simulink model "manipulator_dae"  (R2018b)
settings: Solver=VariableStepAuto  StartTime=0.0  StopTime=10.0  RelTol=1e-3
values from neighbouring files (symbols this model uses):
  alpha_rel = 60*pi/180    (= 1.0471975512)    [parameters.m]
  kp1 = 160    [parameters.m]
  kp2 = 60    [parameters.m]
  kv1 = 11    [parameters.m]
  kv2 = 1.1    [parameters.m]
  rad_deg = 180/pi    (= 57.2957795131)    [parameters.m]
undefined symbols (not defined in the file or in its folder): sys_phdae
settings Model: Creator=a.brugnoli  LastModifiedBy=a.brugnoli

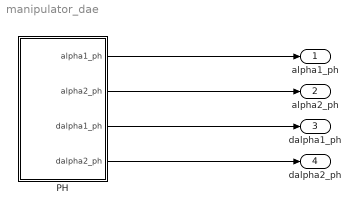
== system manipulator_dae ==
  PH : Subsystem
  alpha1_ph : Outport
  alpha2_ph : Outport  Port=2
  dalpha1_ph : Outport  Port=3
  dalpha2_ph : Outport  Port=4
  wires:
  PH/1(alpha1_ph) -> alpha1_ph/1
  PH/2(alpha2_ph) -> alpha2_ph/1
  PH/4(dalpha2_ph) -> dalpha2_ph/1
  PH/3(dalpha1_ph) -> dalpha1_ph/1

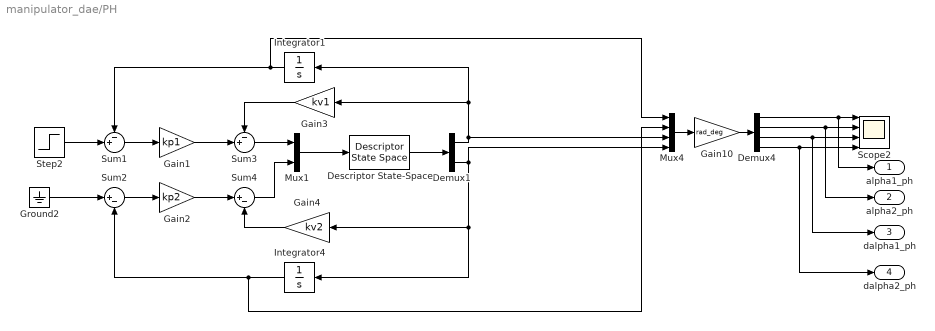
== system manipulator_dae/PH ==
  Demux1 : Demux  Outputs=2
  Demux4 : Demux
  Descriptor State-Space : DescriptorStateSpace  E=sys_phdae.E  A=sys_phdae.A  B=sys_phdae.B  C=sys_phdae.B'  D=0
  Gain1 : Gain  Gain=kp1
  Gain10 : Gain  Gain=rad_deg
  Gain2 : Gain  Gain=kp2
  Gain3 : Gain  Gain=kv1
  Gain4 : Gain  Gain=kv2
  Ground2 : Ground
  Integrator1 : Integrator
  Integrator4 : Integrator
  Mux1 : Mux  Inputs=2
  Mux4 : Mux
  Scope2 : Scope  NumInputPorts=4
  Step2 : Step  After=alpha_rel  SampleTime=0
  Sum1 : Sum  Inputs=-+|
  Sum2 : Sum  Inputs=|+-
  Sum3 : Sum  Inputs=-+|
  Sum4 : Sum  Inputs=|+-
  alpha1_ph : Outport
  alpha2_ph : Outport  Port=2
  dalpha1_ph : Outport  Port=3
  dalpha2_ph : Outport  Port=4
  wires:
  Gain1/1 -> Sum3/2
  Mux4/1 -> Gain10/1
  Gain3/1 -> Sum3/1
  Gain2/1 -> Sum4/1
  Demux4/1 -> alpha1_ph/1, Scope2/1
  Gain10/1 -> Demux4/1
  Sum2/1 -> Gain2/1
  Ground2/1 -> Sum2/1
  Sum1/1 -> Gain1/1
  Demux4/4 -> dalpha2_ph/1, Scope2/4
  Demux1/2 -> Integrator4/1, Gain4/1, Mux4/4
  Demux4/2 -> alpha2_ph/1, Scope2/2
  Integrator1/1 -> Mux4/1, Sum1/1
  Integrator4/1 -> Mux4/2, Sum2/2
  Step2/1 -> Sum1/2
  Demux1/1 -> Gain3/1, Integrator1/1, Mux4/3
  Mux1/1 -> Descriptor State-Space/1
  Demux4/3 -> dalpha1_ph/1, Scope2/3
  Sum4/1 -> Mux1/2
  Sum3/1 -> Mux1/1
  Descriptor State-Space/1 -> Demux1/1
  Gain4/1 -> Sum4/2
